simulink model "hvac_1zone_TCH"  (R2021a)
settings: Solver=FixedStepDiscrete  StartTime=0.0  StopTime=Inf  FixedStep=60  RelTol=1e-3  EnableMultiTasking=on
values from neighbouring files (symbols this model uses):
  beta = 0.08    [main_1zone_td3.m]
  high = 25    [main_1zone_td3.m]
  low = 22    [main_1zone_td3.m]
  Ts = 60*1    (= 60)    [main_1zone_td3.m]
  Ts2 = 60*10    (= 600)    [main_1zone_td3.m]
undefined symbols (not defined in the file or in its folder): ci, CO2_max, id, params, params1, rl
libraries: simulink x6, dspmathops x2, rllib x1
settings Model: Creator=User  LastModifiedBy=diego
settings SolverCC: AlgebraicLoopSolver=TrustRegion
settings DataIOCC: LimitDataPoints=on  SaveFormat=Array  SignalLoggingSaveFormat=ModelDataLogs  SaveOutput=off  SaveTime=off
settings OptimizationCC: LifeSpan=inf
settings DebuggingCC: AlgebraicLoopMsg=none  ArtificialAlgebraicLoopMsg=none  SignalResolutionControl=None  InheritedTsInSrcMsg=none  MultiTaskDSMMsg=none  MultiTaskCondExecSysMsg=none  MultiTaskRateTransMsg=warning  TasksWithSamePriorityMsg=none  SigSpecEnsureSampleTimeMsg=none  IntegerOverflowMsg=none  Int32ToFloatConvMsg=none  ParameterPrecisionLossMsg=none  ParameterTunabilityLossMsg=none  UnconnectedInputMsg=none  UnconnectedOutputMsg=none  UnconnectedLineMsg=none  BusObjectLabelMismatch=none  RootOutportRequireBusObject=none  AllowSymbolicDim=off  UnknownTsInhSupMsg=none  ModelReferenceDataLoggingMessage=none  OperatingPointInterfaceChecksumMismatchMsg=none  SFUnusedDataAndEventsDiag=none  SFUnexpectedBacktrackingDiag=none  SFInvalidInputDataAccessInChartInitDiag=none  SFNoUnconditionalDefaultTransitionDiag=none  SFTransitionOutsideNaturalParentDiag=none  SFUnreachableExecutionPathDiag=none  SFUndirectedBroadcastEventsDiag=none  SFTransitionActionBeforeConditionDiag=none  SFTemporalDelaySmallerThanSampleTimeDiag=none  SFSelfTransitionDiag=none  SFExecutionAtInitializationDiag=none  SFMachineParentedDataDiag=none  IntegerSaturationMsg=none  ArithmeticOperatorsInVariantConditions=warning
settings HardwareCC: ProdBitPerPointer=32  ProdBitPerSizeT=32  ProdBitPerPtrDiffT=32  ProdLargestAtomicFloat=None  ProdIntDivRoundTo=Undefined  ProdEndianess=Unspecified  ProdWordSize=32  ProdHWDeviceType=32-bit Generic
settings ModelReferenceCC: PropagateSignalLabelsOutOfModel=off
settings SFSimCC: SimUseLocalCustomCode=off  CustomCodeUndefinedFunction=UseInterfaceOnly  SimTargetLang=C++
settings RTWCC: RTWUseLocalCustomCode=off
settings CodeAppCC: StateflowObjectComments=on
settings GRTTargetCC: TargetLangStandard=C89/C90 (ANSI)
settings ConfigComp: CovMetricSettings=dw  CovSaveCumulativeToWorkspaceVar=on  CovSaveSingleToWorkspaceVar=on  CovExternalEMLEnable=off

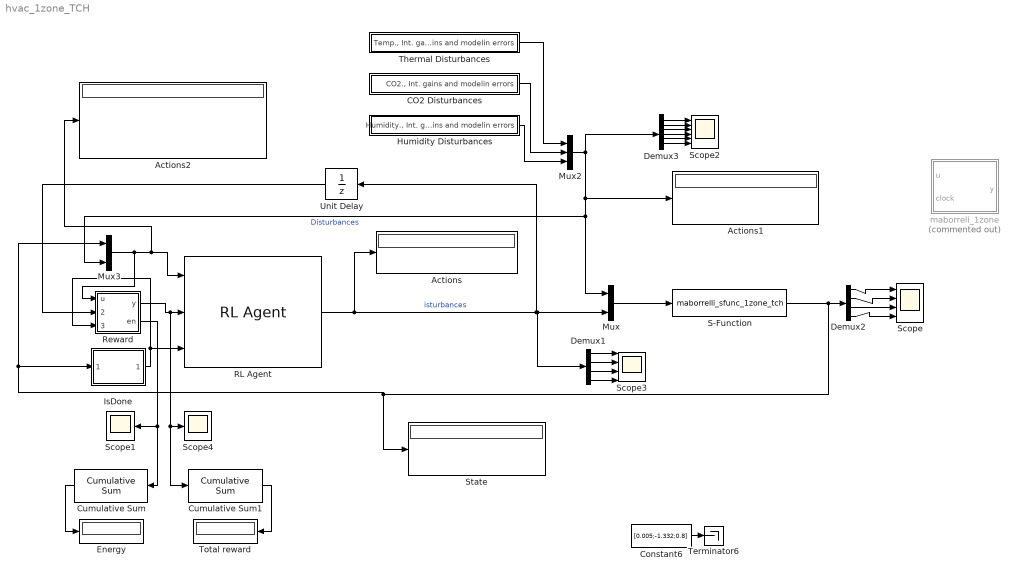
== system hvac_1zone_TCH ==
  Actions : Display
  Actions1 : Display
  Actions2 : Display
  CO2 Disturbances : Subsystem  TreatAsAtomicUnit=on
  Constant6 : Constant  Value=[0.005;-1.332;0.8]
  Cumulative Sum : dspmathops/Cumulative Sum  dim=Channels (running sum)  InputProcessing=Columns as channels (frame based)  reset_popup=None  roundingMode=Floor  overflowMode=off  outputDataTypeStr=Inherit: Same as accumulator  outputMin=[]  outputMax=[]  outputLastDataTypeStr=Inherit: Same as accumulator
  Cumulative Sum1 : dspmathops/Cumulative Sum  dim=Channels (running sum)  InputProcessing=Columns as channels (frame based)  reset_popup=None  roundingMode=Floor  overflowMode=off  outputDataTypeStr=Inherit: Same as accumulator  outputMin=[]  outputMax=[]  outputLastDataTypeStr=Inherit: Same as accumulator
  Demux1 : Demux
  Demux2 : Demux
  Demux3 : Demux  Outputs=6
  Energy : Display
  Humidity Disturbances : Subsystem  TreatAsAtomicUnit=on
  IsDone : MATLAB Function  TreatAsAtomicUnit=on  SystemSampleTime=Ts2
  Mux : Mux  Inputs=2
  Mux2 : Mux  Inputs=3
  Mux3 : Mux  Inputs=2
  RL Agent : rllib/RL Agent  Agent=rl.util.PolicyInstance.get('hvac_1zone_TCH/RL Agent')  ExternalActionAsInput=off  ProvideCumRwd=off  TreatAsDirectFeedthrough=on
  Reward : MATLAB Function  TreatAsAtomicUnit=on  SystemSampleTime=Ts2
  S-Function : S-Function  FunctionName=maborrelli_sfunc_1zone_tch  Parameters=ci,params1,Ts  SFunctionDeploymentMode=off  EnableBusSupport=off
  Scope : Scope  NumInputPorts=4
  Scope1 : Scope
  Scope2 : Scope  NumInputPorts=6
  Scope3 : Scope  NumInputPorts=4
  Scope4 : Scope
  State : Display
  Terminator6 : Terminator
  Thermal Disturbances : Subsystem  TreatAsAtomicUnit=on
  Total reward : Display
  Unit Delay : UnitDelay  SampleTime=Ts2  HasFrameUpgradeWarning=on
  maborreli_1zone : MATLAB Function  Commented=on  TreatAsAtomicUnit=on  SystemSampleTime=Ts
  wires:
  Mux2/1 -> Demux3/1, Actions1/1, Mux3/2, Mux/1  "Disturbances"
  Mux/1 -> S-Function/1
  Constant6/1 -> Terminator6/1
  IsDone/1(value) -> Reward/3(isDone), RL Agent/3
  Reward/1(y) -> RL Agent/2, Cumulative Sum1/1, Scope4/1
  Demux1/2 -> Scope3/2
  Demux1/1 -> Scope3/1
  Demux1/3 -> Scope3/3
  Demux2/1 -> Scope/1
  S-Function/1 -> Mux3/1, IsDone/1(states), State/1, Demux2/1
  RL Agent/1 -> Demux1/1, Mux/2, Unit Delay/1, Actions/1  "isturbances"
  Unit Delay/1 -> Reward/2(actions)
  Mux3/1 -> Reward/1(u), Actions2/1, RL Agent/1
  ? -> maborreli_1zone/2(clock)
  Reward/2(en) -> Cumulative Sum/1, Scope1/1
  Cumulative Sum/1 -> Energy/1
  Thermal Disturbances/1("Temp., Int. gains and modelin errors") -> Mux2/1
  CO2 Disturbances/1("CO2., Int. gains and modelin errors") -> Mux2/2
  Demux1/4 -> Scope3/4
  Demux2/2 -> Scope/2
  Demux3/1 -> Scope2/1
  Demux3/2 -> Scope2/2
  Demux3/3 -> Scope2/3
  Demux3/4 -> Scope2/4
  Humidity Disturbances/1("Humidity., Int. gains and modelin errors") -> Mux2/3
  Demux3/5 -> Scope2/5
  Demux3/6 -> Scope2/6
  Demux2/3 -> Scope/3
  Demux2/4 -> Scope/4
  Cumulative Sum1/1 -> Total reward/1

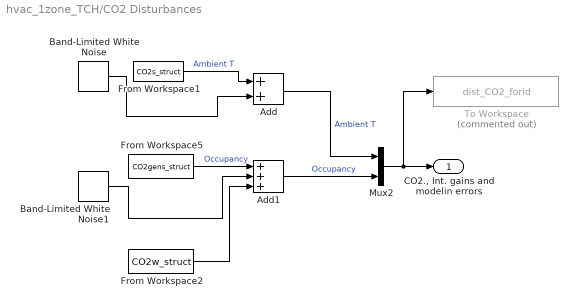
== system hvac_1zone_TCH/CO2 Disturbances ==
  Add : Sum
  Add1 : Sum  Inputs=+++
  Band-Limited White Noise : simulink/Sources/Band-Limited White Noise  Cov=0  Ts=3600  seed=[23341]
  Band-Limited White Noise1 : simulink/Sources/Band-Limited White Noise  Cov=0  Ts=3600  seed=[23341]
  From Workspace1 : FromWorkspace  VariableName=CO2s_struct  OutDataTypeStr=double  SampleTime=Ts  ZeroCross=off
  From Workspace2 : FromWorkspace  VariableName=CO2w_struct  OutDataTypeStr=double  SampleTime=Ts  ZeroCross=off
  From Workspace5 : FromWorkspace  VariableName=CO2gens_struct  OutDataTypeStr=double  SampleTime=Ts  ZeroCross=off
  Mux2 : Mux  Inputs=2
  To Workspace : ToWorkspace  Commented=on  VariableName=dist_CO2_forid  SaveFormat=Timeseries  SampleTime=id.Delta
  "CO2., Int. gains and modelin errors" : Outport
  wires:
  From Workspace1/1 -> Add/1  "Ambient T"
  Band-Limited White Noise/1 -> Add/2
  Add/1 -> Mux2/1  "Ambient T"
  From Workspace5/1 -> Add1/1  "Occupancy"
  Band-Limited White Noise1/1 -> Add1/2
  From Workspace2/1 -> Add1/3
  Mux2/1 -> To Workspace/1, "CO2., Int. gains and modelin errors"/1
  Add1/1 -> Mux2/2  "Occupancy"

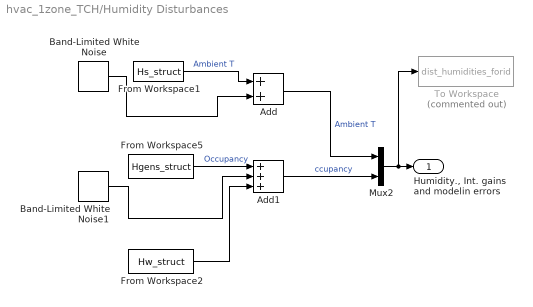
== system hvac_1zone_TCH/Humidity Disturbances ==
  Add : Sum
  Add1 : Sum  Inputs=+++
  Band-Limited White Noise : simulink/Sources/Band-Limited White Noise  Cov=0  Ts=3600  seed=[23341]
  Band-Limited White Noise1 : simulink/Sources/Band-Limited White Noise  Cov=0  Ts=3600  seed=[23341]
  From Workspace1 : FromWorkspace  VariableName=Hs_struct  OutDataTypeStr=double  SampleTime=Ts  ZeroCross=off
  From Workspace2 : FromWorkspace  VariableName=Hw_struct  OutDataTypeStr=double  SampleTime=Ts  ZeroCross=off
  From Workspace5 : FromWorkspace  VariableName=Hgens_struct  OutDataTypeStr=double  SampleTime=Ts  ZeroCross=off
  Mux2 : Mux  Inputs=2
  To Workspace : ToWorkspace  Commented=on  VariableName=dist_humidities_forid  SaveFormat=Timeseries  SampleTime=id.Delta
  "Humidity., Int. gains and modelin errors" : Outport
  wires:
  From Workspace1/1 -> Add/1  "Ambient T"
  Band-Limited White Noise/1 -> Add/2
  Add/1 -> Mux2/1  "Ambient T"
  From Workspace5/1 -> Add1/1  "Occupancy"
  Band-Limited White Noise1/1 -> Add1/2
  From Workspace2/1 -> Add1/3
  Mux2/1 -> To Workspace/1, "Humidity., Int. gains and modelin errors"/1
  Add1/1 -> Mux2/2  "ccupancy"

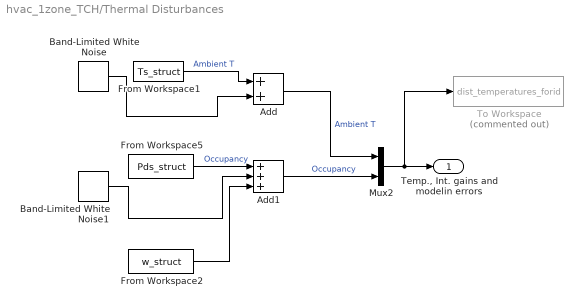
== system hvac_1zone_TCH/Thermal Disturbances ==
  Add : Sum
  Add1 : Sum  Inputs=+++
  Band-Limited White Noise : simulink/Sources/Band-Limited White Noise  Cov=1.5  Ts=3600  seed=[23341]
  Band-Limited White Noise1 : simulink/Sources/Band-Limited White Noise  Cov=0.5  Ts=3600  seed=[23341]
  From Workspace1 : FromWorkspace  VariableName=Ts_struct  OutDataTypeStr=double  SampleTime=Ts  ZeroCross=off
  From Workspace2 : FromWorkspace  VariableName=w_struct  OutDataTypeStr=double  SampleTime=Ts  ZeroCross=off
  From Workspace5 : FromWorkspace  VariableName=Pds_struct  OutDataTypeStr=double  SampleTime=Ts  ZeroCross=off
  Mux2 : Mux  Inputs=2
  To Workspace : ToWorkspace  Commented=on  VariableName=dist_temperatures_forid  SaveFormat=Timeseries  SampleTime=id.Delta
  "Temp., Int. gains and modelin errors" : Outport
  wires:
  Add1/1 -> Mux2/2  "Occupancy"
  From Workspace1/1 -> Add/1  "Ambient T"
  Band-Limited White Noise/1 -> Add/2
  Add/1 -> Mux2/1  "Ambient T"
  From Workspace5/1 -> Add1/1  "Occupancy"
  Band-Limited White Noise1/1 -> Add1/2
  From Workspace2/1 -> Add1/3
  Mux2/1 -> To Workspace/1, "Temp., Int. gains and modelin errors"/1

== matlab function hvac_1zone_TCH/IsDone ==
  data: states input; value output
function value = fcn(states)
 low = -0;
 max = 50;
 value = 0; 
 %disp(length(block.InputPort(1).Data))
 for i=1:length(states)
     %disp(i)
     if i == 3
         break
     end
     if states(3)>(3200*1e-6)
         value = 1;
         break
     end
     aux = states(i);
     %disp(aux)
     if (aux < low || aux > max) 
        %disp(abs(aux - low))
        value = 1;
        break
     end
     %disp('if3')
 end

== matlab function hvac_1zone_TCH/Reward ==
  data: u input; y output; actions input; isDone input; low parameter; high parameter; beta parameter; en output; params parameter; CO2_max parameter
function [y, en] = reward(u ,  actions, isDone, low, high, beta, params, CO2_max)
 ms = actions(1);
 Dt = actions(2);
 Dth = actions(3);
 delta = actions(4);
 reward = 0;
 cp = params.cp;
 eta = params.eta;
 kf = params.kf;
 eta_h = params.eta_h;
 %mr = delta*u_1(1)+(1-delta)*u_1(4);
 %Añadir energía:
 e = (kf*(ms)^2)/1000;
 e = e + ((-cp/eta)*ms*(Dt))/1000;
 for i=1:1
     aux = u(1);
     e = e + ((cp/eta_h)*ms*(Dth - Dt))/1000;
     if ms == 0 && Dth~=0
         reward = reward - 10;
     end
     if ms == 0 && Dt~=0
         reward = reward - 1;
     end
     %disp('estado')
     %disp(aux)
     if (aux < low || aux > high)
        reward = reward - 0.8*(min(abs(aux - low), abs(aux - high))+ (min( abs(aux - low), abs(aux - high)))^2);
     end
     
     if CO2_max < u(3)
        %disp(-abs(CO2_max - u(3))*10000)
        reward = reward - abs(CO2_max - u(3))*20000;
     end
     Hum = u(5);
     %disp(Hum)
     if (0.35 > Hum) || (Hum > 0.65)
         reward = reward - 5*min(abs(Hum-0.35),abs(Hum-0.65));
         %disp(min(abs(Hum-0.35),abs(Hum-0.65))*7)
     end
     %Entregar bonificación por estar en el estado
     %if (aux >= low && aux <= high)
     %    reward = reward + 1;
     %end
 reward = reward -beta* e; 
 en = e;
 end
 if isDone
     reward = -2000;
 end
y = reward;

== matlab function hvac_1zone_TCH/maborreli_1zone ==
  data: u input; y output; params1 parameter; ci parameter; Ts parameter; states data_store_memory; clock input
function y = fcn(u,params1, ci, Ts, clock)
ST = Ts;
params = params1;
global states;
dT = [0;0];
delta=u(5);
if clock == 0
    dT = ci;
else
    x = states;
    dT(1)=x(1)+(ST*u(3)*params.cp*((delta*x(1)+(1-delta)*u(1)+u(4))-x(1))+ ST*(x(2)-x(1))/params.R+...
        ST*(u(1)-x(1))/params.Roa+ST*u(2))/params.C1;
    dT(2)=x(2)+ST*(x(1)-x(2))/params.R/params.C2;
end
states = dT;
y = dT;
